simulink model "labc2_ackerman_funcionando"  (R2023a)
settings: Solver=VariableStepAuto  StartTime=0.0  StopTime=10.0  RelTol=1e-3
values from neighbouring files (symbols this model uses):
  A = [-Ra/La -kg/La/kt; ka*kt/J -f/J]    [labc2_p2_final.m]    (also in robusto2_lc2.m = [[ -113.5203 -34.3792];[27.0249 -0.3312]]; robusto_labc2.m = [[ -113.5203 -34.3792];[27.0249 -0.3312]])
  b = [1/La;0]    [labc2_p2_final.m]    (also in robusto2_lc2.m = [46.6079 0]'; robusto_labc2.m = [46.6079 0]')
  c = [0 1]    [labc2_p2_final.m]    (also in robusto2_lc2.m; robusto_labc2.m)
  kt_ee = place(A, b, polos)    [labc2_p2_final.m]    (also in robusto2_lc2.m = k_robusto(1:2); robusto_labc2.m)
settings Model: Creator=wesle  LastModifiedBy=wesle

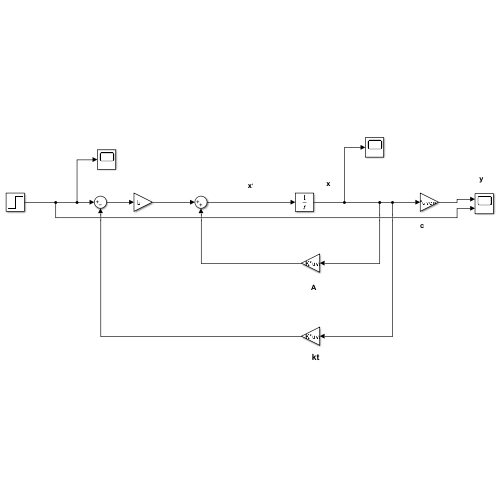
[thumbnail: Simulink's stored preview of the top-level diagram]
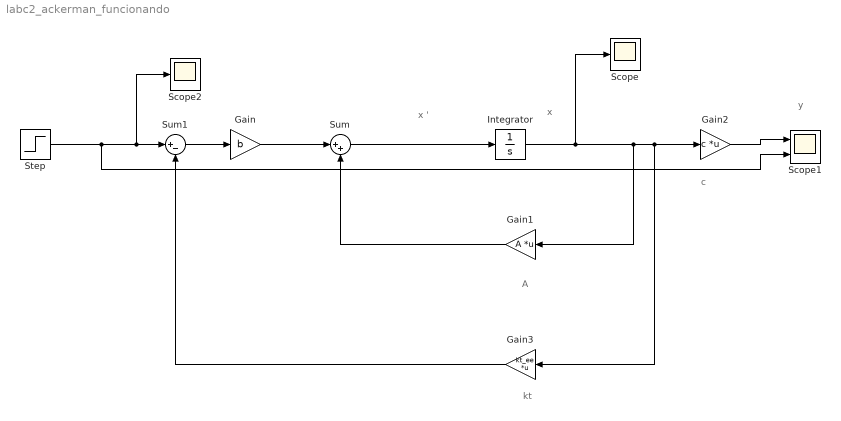
== system labc2_ackerman_funcionando ==
  note: kt
  note: c
  note: A
  note: x '
  note: x
  note: y
  Gain : Gain  Gain=b
  Gain1 : Gain  Gain=A  Multiplication=Matrix(K*u) (u vector)
  Gain2 : Gain  Gain=c  Multiplication=Matrix(K*u) (u vector)
  Gain3 : Gain  Gain=kt_ee  Multiplication=Matrix(K*u) (u vector)
  Integrator : Integrator
  Scope : Scope
  Scope1 : Scope  NumInputPorts=2
  Scope2 : Scope
  Step : Step  SampleTime=0
  Sum : Sum  Inputs=|++
  Sum1 : Sum  Inputs=|+-
  wires:
  Sum/1 -> Integrator/1
  Gain/1 -> Sum/1
  Gain1/1 -> Sum/2
  Step/1 -> Scope1/2, Sum1/1, Scope2/1
  Integrator/1 -> Scope/1, Gain1/1, Gain3/1, Gain2/1
  Gain2/1 -> Scope1/1
  Gain3/1 -> Sum1/2
  Sum1/1 -> Gain/1
